simulink model "OMAP_ver_MIL10"  (R2018b)
settings: Solver=FixedStepDiscrete  StartTime=0.0  StopTime=10.0  FixedStep=0.01  RelTol=1e-3
undefined symbols (not defined in the file or in its folder): OMAP_Switch_EMS, OMAP_Switch_EPS, OMAP_Switch_ESC, OMAP_Switch_IC, OMAP_Switch_OTHER, TH_HMIClb_tiDgrdIconWarnHiDurT_C, TH_HMIClb_tiDgrdIconWarnLoDurT_C, TH_HMIClb_tiDgrdVocWarnDurT_C, TH_HMIClb_tiHndOffTxtWarnT_C, TH_HMIClb_tiHndOffVocWarnT_C, TH_HMIClb_tiSWALimFlgDetT_C, TH_HMIClb_tiTxtLimT_C
libraries: simulink x118
(part 8 of 9)

== system OMAP_ver_MIL10/OMAP_Module/ICA_Direct_G59/ICA_Define/Subsystem1/Dspl/DsplPrcs/Txt/TxtOff ==
  TxtOff_stTHState : Inport
  TxtOff_stLstTHState : Inport  Port=2
  Constant1 : Constant  OutDataTypeStr=uint16
  Constant2 : Constant  Value=0  OutDataTypeStr=uint16
  Hold : Subsystem  TreatAsAtomicUnit=on
  If : If  NumInputs=2  IfExpression=u1 == 0 & u2 ~= 0 & u2 ~= 5  ElseIfExpressions=u1 ~= 0
  Merge : Merge  Inputs=3
  Start : Subsystem  TreatAsAtomicUnit=on
  Stop : Subsystem  TreatAsAtomicUnit=on
  Unit Delay1 : UnitDelay  SampleTime=-1
  TxtOff_stOff : Outport
  wires:
  TxtOff_stTHState/1 -> If/1
  Merge/1 -> Unit Delay1/1, TxtOff_stOff/1
  Start/1(Out1) -> Merge/1
  TxtOff_stLstTHState/1 -> If/2
  Constant1/1 -> Start/1(In1)
  If/1 -> Start/Action
  Constant2/1 -> Stop/1(In1)
  If/2 -> Stop/Action
  Unit Delay1/1 -> Hold/1(In1)
  If/3 -> Hold/Action
  Stop/1(Out1) -> Merge/2
  Hold/1(Out1) -> Merge/3

== system OMAP_ver_MIL10/OMAP_Module/ICA_Direct_G59/ICA_Define/Subsystem1/Dspl/DsplPrcs/Txt/TxtOffToFault ==
  TxtOffToFault_stTHState : Inport
  TxtOffToFault_stLstTHState : Inport  Port=2
  TxtOffToFault_stACCState : Inport  Port=3
  Constant1 : Constant  OutDataTypeStr=uint16
  Constant2 : Constant  Value=0  OutDataTypeStr=uint16
  Hold : Subsystem  TreatAsAtomicUnit=on
  If : If  NumInputs=3  IfExpression=u1 == 5 & u2 == 0 & u3 ~= 15  ElseIfExpressions=u1 ~= 5 | u3 == 15
  Merge : Merge  Inputs=3
  Start : Subsystem  TreatAsAtomicUnit=on
  Stop : Subsystem  TreatAsAtomicUnit=on
  Unit Delay1 : UnitDelay  SampleTime=-1
  TxtOffToFault_stOffToFault : Outport
  wires:
  TxtOffToFault_stTHState/1 -> If/1
  Merge/1 -> Unit Delay1/1, TxtOffToFault_stOffToFault/1
  Start/1(Out1) -> Merge/1
  TxtOffToFault_stLstTHState/1 -> If/2
  TxtOffToFault_stACCState/1 -> If/3
  Constant1/1 -> Start/1(In1)
  If/1 -> Start/Action
  Constant2/1 -> Stop/1(In1)
  If/2 -> Stop/Action
  Unit Delay1/1 -> Hold/1(In1)
  If/3 -> Hold/Action
  Stop/1(Out1) -> Merge/2
  Hold/1(Out1) -> Merge/3

== system OMAP_ver_MIL10/OMAP_Module/ICA_Direct_G59/ICA_Define/Subsystem1/Dspl/DsplPrcs/Txt/TxtOn ==
  TxtOn_stTHState : Inport
  TxtOn_stLstTHState : Inport  Port=2
  Constant1 : Constant  OutDataTypeStr=uint16
  Constant2 : Constant  Value=0  OutDataTypeStr=uint16
  Hold : Subsystem  TreatAsAtomicUnit=on
  If : If  NumInputs=2  IfExpression=u1 == 8 & u2 == 0  ElseIfExpressions=u1 == 0 | u1 == 5
  Merge : Merge  Inputs=3
  Start : Subsystem  TreatAsAtomicUnit=on
  Stop : Subsystem  TreatAsAtomicUnit=on
  Unit Delay1 : UnitDelay  SampleTime=-1
  TxtOn_stOn : Outport
  wires:
  TxtOn_stTHState/1 -> If/1
  Merge/1 -> Unit Delay1/1, TxtOn_stOn/1
  Start/1(Out1) -> Merge/1
  TxtOn_stLstTHState/1 -> If/2
  Constant1/1 -> Start/1(In1)
  If/1 -> Start/Action
  Constant2/1 -> Stop/1(In1)
  If/2 -> Stop/Action
  Unit Delay1/1 -> Hold/1(In1)
  If/3 -> Hold/Action
  Stop/1(Out1) -> Merge/2
  Hold/1(Out1) -> Merge/3

== system OMAP_ver_MIL10/OMAP_Module/ICA_Direct_G59/ICA_Define/Subsystem1/Dspl/DsplPrcs/Txt/TxtOnToFault ==
  TxtOnToFault_stTHState : Inport
  TxtOnToFault_stLstTHState : Inport  Port=2
  Constant1 : Constant  OutDataTypeStr=uint16
  Constant2 : Constant  Value=0  OutDataTypeStr=uint16
  Hold : Subsystem  TreatAsAtomicUnit=on
  If : If  NumInputs=2  IfExpression=u1 == 5 & u2 ~= 0 & u2 ~= 5  ElseIfExpressions=u1 ~= 5
  Merge : Merge  Inputs=3
  Start : Subsystem  TreatAsAtomicUnit=on
  Stop : Subsystem  TreatAsAtomicUnit=on
  Unit Delay1 : UnitDelay  SampleTime=-1
  TxtOnToFault_stOnToFault : Outport
  wires:
  Hold/1(Out1) -> Merge/3
  Stop/1(Out1) -> Merge/2
  If/3 -> Hold/Action
  Unit Delay1/1 -> Hold/1(In1)
  If/2 -> Stop/Action
  Constant2/1 -> Stop/1(In1)
  If/1 -> Start/Action
  Constant1/1 -> Start/1(In1)
  TxtOnToFault_stLstTHState/1 -> If/2
  Start/1(Out1) -> Merge/1
  Merge/1 -> TxtOnToFault_stOnToFault/1, Unit Delay1/1
  TxtOnToFault_stTHState/1 -> If/1

== system OMAP_ver_MIL10/OMAP_Module/ICA_Direct_G59/ICA_Define/Subsystem1/Dspl/DsplPrcs/Txt/Txt_Tlimit ==
  incrcondition : Inport
  maxlimit : Inport  Port=2
  Compare To Constant : simulink/Logic and Bit Operations/Compare To Constant  relop===  const=boolean(1)  OutDataTypeStr=boolean
  Compare To Constant1 : simulink/Logic and Bit Operations/Compare To Constant  relop===  const=uint16(0)  OutDataTypeStr=boolean
  Constant : Constant  Value=0  OutDataTypeStr=uint16
  Constant1 : Constant  Value=0  OutDataTypeStr=uint16
  Constant2 : Constant  OutDataTypeStr=uint16
  Constant4 : Constant  OutDataTypeStr=uint16
  Constant5 : Constant  Value=0  OutDataTypeStr=uint16
  Data Type Conversion3 : DataTypeConversion  OutDataTypeStr=uint16
  Detect Fall Nonpositive : simulink/Logic and Bit Operations/Detect Fall Nonpositive  vinit=0  OutDataTypeStr=boolean
      settings: SourceProductName=Simulink  SourceProductBaseCode=SL
  Detect Rise Positive : simulink/Logic and Bit Operations/Detect Rise Positive  vinit=0  OutDataTypeStr=boolean
  Hold : Subsystem  TreatAsAtomicUnit=on
  If : If  NumInputs=3  IfExpression=u1 == 1  ElseIfExpressions=u2 == 1 | u3 == 1
  Logical Operator : Logic  Operator=OR  AllPortsSameDT=off  OutDataTypeStr=boolean
  Merge : Merge  Inputs=3
  MinMax1 : MinMax  Inputs=2  OutDataTypeStr=uint16  InputSameDT=on
  Relational Operator : RelationalOperator  Operator=<=  OutDataTypeStr=boolean  RndMeth=Nearest
  Start : Subsystem  TreatAsAtomicUnit=on
  Stop : Subsystem  TreatAsAtomicUnit=on
  Sum : Sum  OutDataTypeStr=Inherit: Inherit via back propagation  InputSameDT=on
  Unit Delay : UnitDelay  SampleTime=-1
  Unit Delay1 : UnitDelay  SampleTime=-1
  Unit Delay3 : UnitDelay  SampleTime=-1
  inc switch : Switch  Criteria=u2 ~= 0  Threshold=1  OutDataTypeStr=Inherit: Inherit via back propagation  InputSameDT=on
  reset switch : Switch  Criteria=u2 ~= 0  Threshold=1  OutDataTypeStr=Inherit: Inherit via back propagation  InputSameDT=on
  counter_status : Outport
  counter_reset : Outport  Port=2
  wires:
  Unit Delay/1 -> Sum/2
  maxlimit/1 -> Relational Operator/1, MinMax1/2
  MinMax1/1 -> reset switch/3
  Hold/1(Out1) -> Merge/3
  Unit Delay1/1 -> Hold/1(In1)
  If/3 -> Hold/Action
  Stop/1(Out1) -> Merge/2
  Constant4/1 -> Start/1(In1)
  If/1 -> Start/Action
  Start/1(Out1) -> Merge/1
  If/2 -> Stop/Action
  Constant5/1 -> Stop/1(In1)
  incrcondition/1 -> Detect Rise Positive/1, Detect Fall Nonpositive/1
  Detect Rise Positive/1 -> If/1
  Detect Fall Nonpositive/1 -> If/2
  Sum/1 -> MinMax1/1
  reset switch/1 -> Relational Operator/2, Unit Delay/1
  Constant1/1 -> reset switch/1
  Relational Operator/1 -> Unit Delay3/1
  [reset] -> If/3
  [reset] -> Compare To Constant/1
  Constant2/1 -> inc switch/1
  Constant/1 -> inc switch/3
  inc switch/1 -> Sum/1
  Logical Operator/1 -> reset switch/2
  Data Type Conversion3/1 -> counter_reset/1
  Unit Delay3/1 -> Data Type Conversion3/1, [reset]
  Compare To Constant/1 -> Logical Operator/2
  Merge/1 -> Compare To Constant1/1, counter_status/1, inc switch/2, Unit Delay1/1
  Compare To Constant1/1 -> Logical Operator/1

== system OMAP_ver_MIL10/OMAP_Module/ICA_Direct_G59/ICA_Define/Subsystem1/Dspl/DsplPrcs/Txt/Txt_Tlimit1 ==
  incrcondition : Inport
  maxlimit : Inport  Port=2
  Compare To Constant : simulink/Logic and Bit Operations/Compare To Constant  relop===  const=boolean(1)  OutDataTypeStr=boolean
  Compare To Constant1 : simulink/Logic and Bit Operations/Compare To Constant  relop===  const=uint16(0)  OutDataTypeStr=boolean
  Constant : Constant  Value=0  OutDataTypeStr=uint16
  Constant1 : Constant  Value=0  OutDataTypeStr=uint16
  Constant2 : Constant  OutDataTypeStr=uint16
  Constant4 : Constant  OutDataTypeStr=uint16
  Constant5 : Constant  Value=0  OutDataTypeStr=uint16
  Data Type Conversion3 : DataTypeConversion  OutDataTypeStr=uint16
  Detect Fall Nonpositive : simulink/Logic and Bit Operations/Detect Fall Nonpositive  vinit=0  OutDataTypeStr=boolean
      settings: SourceProductName=Simulink  SourceProductBaseCode=SL
  Detect Rise Positive : simulink/Logic and Bit Operations/Detect Rise Positive  vinit=0  OutDataTypeStr=boolean
  Hold : Subsystem  TreatAsAtomicUnit=on
  If : If  NumInputs=3  IfExpression=u1 == 1  ElseIfExpressions=u2 == 1 | u3 == 1
  Logical Operator : Logic  Operator=OR  AllPortsSameDT=off  OutDataTypeStr=boolean
  Merge : Merge  Inputs=3
  MinMax1 : MinMax  Inputs=2  OutDataTypeStr=uint16  InputSameDT=on
  Relational Operator : RelationalOperator  Operator=<=  OutDataTypeStr=boolean  RndMeth=Nearest
  Start : Subsystem  TreatAsAtomicUnit=on
  Stop : Subsystem  TreatAsAtomicUnit=on
  Sum : Sum  OutDataTypeStr=Inherit: Inherit via back propagation  InputSameDT=on
  Unit Delay : UnitDelay  SampleTime=-1
  Unit Delay1 : UnitDelay  SampleTime=-1
  Unit Delay3 : UnitDelay  SampleTime=-1
  inc switch : Switch  Criteria=u2 ~= 0  Threshold=1  OutDataTypeStr=Inherit: Inherit via back propagation  InputSameDT=on
  reset switch : Switch  Criteria=u2 ~= 0  Threshold=1  OutDataTypeStr=Inherit: Inherit via back propagation  InputSameDT=on
  counter_status : Outport
  counter_reset : Outport  Port=2
  wires:
  Compare To Constant1/1 -> Logical Operator/1
  Merge/1 -> Unit Delay1/1, inc switch/2, counter_status/1, Compare To Constant1/1
  Compare To Constant/1 -> Logical Operator/2
  Unit Delay3/1 -> [reset], Data Type Conversion3/1
  Data Type Conversion3/1 -> counter_reset/1
  Logical Operator/1 -> reset switch/2
  inc switch/1 -> Sum/1
  Constant/1 -> inc switch/3
  Constant2/1 -> inc switch/1
  [reset] -> Compare To Constant/1
  [reset] -> If/3
  Relational Operator/1 -> Unit Delay3/1
  Constant1/1 -> reset switch/1
  reset switch/1 -> Unit Delay/1, Relational Operator/2
  Sum/1 -> MinMax1/1
  Detect Fall Nonpositive/1 -> If/2
  Detect Rise Positive/1 -> If/1
  incrcondition/1 -> Detect Fall Nonpositive/1, Detect Rise Positive/1
  Constant5/1 -> Stop/1(In1)
  If/2 -> Stop/Action
  Start/1(Out1) -> Merge/1
  If/1 -> Start/Action
  Constant4/1 -> Start/1(In1)
  Stop/1(Out1) -> Merge/2
  If/3 -> Hold/Action
  Unit Delay1/1 -> Hold/1(In1)
  Hold/1(Out1) -> Merge/3
  MinMax1/1 -> reset switch/3
  maxlimit/1 -> MinMax1/2, Relational Operator/1
  Unit Delay/1 -> Sum/2

== system OMAP_ver_MIL10/OMAP_Module/ICA_Direct_G59/ICA_Define/Subsystem1/Dspl/DsplPrcs/Txt/Txt_Tlimit2 ==
  incrcondition : Inport
  maxlimit : Inport  Port=2
  Compare To Constant : simulink/Logic and Bit Operations/Compare To Constant  relop===  const=boolean(1)  OutDataTypeStr=boolean
  Compare To Constant1 : simulink/Logic and Bit Operations/Compare To Constant  relop===  const=uint16(0)  OutDataTypeStr=boolean
  Constant : Constant  Value=0  OutDataTypeStr=uint16
  Constant1 : Constant  Value=0  OutDataTypeStr=uint16
  Constant2 : Constant  OutDataTypeStr=uint16
  Constant4 : Constant  OutDataTypeStr=uint16
  Constant5 : Constant  Value=0  OutDataTypeStr=uint16
  Data Type Conversion3 : DataTypeConversion  OutDataTypeStr=uint16
  Detect Fall Nonpositive : simulink/Logic and Bit Operations/Detect Fall Nonpositive  vinit=0  OutDataTypeStr=boolean
      settings: SourceProductName=Simulink  SourceProductBaseCode=SL
  Detect Rise Positive : simulink/Logic and Bit Operations/Detect Rise Positive  vinit=0  OutDataTypeStr=boolean
  Hold : Subsystem  TreatAsAtomicUnit=on
  If : If  NumInputs=3  IfExpression=u1 == 1  ElseIfExpressions=u2 == 1 | u3 == 1
  Logical Operator : Logic  Operator=OR  AllPortsSameDT=off  OutDataTypeStr=boolean
  Merge : Merge  Inputs=3
  MinMax1 : MinMax  Inputs=2  OutDataTypeStr=uint16  InputSameDT=on
  Relational Operator : RelationalOperator  Operator=<=  OutDataTypeStr=boolean  RndMeth=Nearest
  Start : Subsystem  TreatAsAtomicUnit=on
  Stop : Subsystem  TreatAsAtomicUnit=on
  Sum : Sum  OutDataTypeStr=Inherit: Inherit via back propagation  InputSameDT=on
  Unit Delay : UnitDelay  SampleTime=-1
  Unit Delay1 : UnitDelay  SampleTime=-1
  Unit Delay3 : UnitDelay  SampleTime=-1
  inc switch : Switch  Criteria=u2 ~= 0  Threshold=1  OutDataTypeStr=Inherit: Inherit via back propagation  InputSameDT=on
  reset switch : Switch  Criteria=u2 ~= 0  Threshold=1  OutDataTypeStr=Inherit: Inherit via back propagation  InputSameDT=on
  counter_status : Outport
  counter_reset : Outport  Port=2
  wires:
  Unit Delay/1 -> Sum/2
  maxlimit/1 -> Relational Operator/1, MinMax1/2
  MinMax1/1 -> reset switch/3
  Hold/1(Out1) -> Merge/3
  Unit Delay1/1 -> Hold/1(In1)
  If/3 -> Hold/Action
  Stop/1(Out1) -> Merge/2
  Constant4/1 -> Start/1(In1)
  If/1 -> Start/Action
  Start/1(Out1) -> Merge/1
  If/2 -> Stop/Action
  Constant5/1 -> Stop/1(In1)
  incrcondition/1 -> Detect Rise Positive/1, Detect Fall Nonpositive/1
  Detect Rise Positive/1 -> If/1
  Detect Fall Nonpositive/1 -> If/2
  Sum/1 -> MinMax1/1
  reset switch/1 -> Relational Operator/2, Unit Delay/1
  Constant1/1 -> reset switch/1
  Relational Operator/1 -> Unit Delay3/1
  [reset] -> If/3
  [reset] -> Compare To Constant/1
  Constant2/1 -> inc switch/1
  Constant/1 -> inc switch/3
  inc switch/1 -> Sum/1
  Logical Operator/1 -> reset switch/2
  Data Type Conversion3/1 -> counter_reset/1
  Unit Delay3/1 -> Data Type Conversion3/1, [reset]
  Compare To Constant/1 -> Logical Operator/2
  Merge/1 -> Compare To Constant1/1, counter_status/1, inc switch/2, Unit Delay1/1
  Compare To Constant1/1 -> Logical Operator/1

== system OMAP_ver_MIL10/OMAP_Module/ICA_Direct_G59/ICA_Define/Subsystem1/Dspl/DsplPrcs/Txt/Txt_Tlimit3 ==
  incrcondition : Inport
  maxlimit : Inport  Port=2
  Compare To Constant : simulink/Logic and Bit Operations/Compare To Constant  relop===  const=boolean(1)  OutDataTypeStr=boolean
  Compare To Constant1 : simulink/Logic and Bit Operations/Compare To Constant  relop===  const=uint16(0)  OutDataTypeStr=boolean
  Constant : Constant  Value=0  OutDataTypeStr=uint16
  Constant1 : Constant  Value=0  OutDataTypeStr=uint16
  Constant2 : Constant  OutDataTypeStr=uint16
  Constant4 : Constant  OutDataTypeStr=uint16
  Constant5 : Constant  Value=0  OutDataTypeStr=uint16
  Data Type Conversion3 : DataTypeConversion  OutDataTypeStr=uint16
  Detect Fall Nonpositive : simulink/Logic and Bit Operations/Detect Fall Nonpositive  vinit=0  OutDataTypeStr=boolean
      settings: SourceProductName=Simulink  SourceProductBaseCode=SL
  Detect Rise Positive : simulink/Logic and Bit Operations/Detect Rise Positive  vinit=0  OutDataTypeStr=boolean
  Hold : Subsystem  TreatAsAtomicUnit=on
  If : If  NumInputs=3  IfExpression=u1 == 1  ElseIfExpressions=u2 == 1 | u3 == 1
  Logical Operator : Logic  Operator=OR  AllPortsSameDT=off  OutDataTypeStr=boolean
  Merge : Merge  Inputs=3
  MinMax1 : MinMax  Inputs=2  OutDataTypeStr=uint16  InputSameDT=on
  Relational Operator : RelationalOperator  Operator=<=  OutDataTypeStr=boolean  RndMeth=Nearest
  Start : Subsystem  TreatAsAtomicUnit=on
  Stop : Subsystem  TreatAsAtomicUnit=on
  Sum : Sum  OutDataTypeStr=Inherit: Inherit via back propagation  InputSameDT=on
  Unit Delay : UnitDelay  SampleTime=-1
  Unit Delay1 : UnitDelay  SampleTime=-1
  Unit Delay3 : UnitDelay  SampleTime=-1
  inc switch : Switch  Criteria=u2 ~= 0  Threshold=1  OutDataTypeStr=Inherit: Inherit via back propagation  InputSameDT=on
  reset switch : Switch  Criteria=u2 ~= 0  Threshold=1  OutDataTypeStr=Inherit: Inherit via back propagation  InputSameDT=on
  counter_status : Outport
  counter_reset : Outport  Port=2
  wires:
  Compare To Constant1/1 -> Logical Operator/1
  Merge/1 -> Unit Delay1/1, inc switch/2, counter_status/1, Compare To Constant1/1
  Compare To Constant/1 -> Logical Operator/2
  Unit Delay3/1 -> [reset], Data Type Conversion3/1
  Data Type Conversion3/1 -> counter_reset/1
  Logical Operator/1 -> reset switch/2
  inc switch/1 -> Sum/1
  Constant/1 -> inc switch/3
  Constant2/1 -> inc switch/1
  [reset] -> Compare To Constant/1
  [reset] -> If/3
  Relational Operator/1 -> Unit Delay3/1
  Constant1/1 -> reset switch/1
  reset switch/1 -> Unit Delay/1, Relational Operator/2
  Sum/1 -> MinMax1/1
  Detect Fall Nonpositive/1 -> If/2
  Detect Rise Positive/1 -> If/1
  incrcondition/1 -> Detect Fall Nonpositive/1, Detect Rise Positive/1
  Constant5/1 -> Stop/1(In1)
  If/2 -> Stop/Action
  Start/1(Out1) -> Merge/1
  If/1 -> Start/Action
  Constant4/1 -> Start/1(In1)
  Stop/1(Out1) -> Merge/2
  If/3 -> Hold/Action
  Unit Delay1/1 -> Hold/1(In1)
  Hold/1(Out1) -> Merge/3
  MinMax1/1 -> reset switch/3
  maxlimit/1 -> MinMax1/2, Relational Operator/1
  Unit Delay/1 -> Sum/2

== system OMAP_ver_MIL10/OMAP_Module/ICA_Direct_G59/ICA_Define/Subsystem1/Dspl/DsplPrcs/Txt/Txt_Tlimit4 ==
  incrcondition : Inport
  maxlimit : Inport  Port=2
  Compare To Constant : simulink/Logic and Bit Operations/Compare To Constant  relop===  const=boolean(1)  OutDataTypeStr=boolean
  Compare To Constant1 : simulink/Logic and Bit Operations/Compare To Constant  relop===  const=uint16(0)  OutDataTypeStr=boolean
  Constant : Constant  Value=0  OutDataTypeStr=uint16
  Constant1 : Constant  Value=0  OutDataTypeStr=uint16
  Constant2 : Constant  OutDataTypeStr=uint16
  Constant4 : Constant  OutDataTypeStr=uint16
  Constant5 : Constant  Value=0  OutDataTypeStr=uint16
  Data Type Conversion3 : DataTypeConversion  OutDataTypeStr=uint16
  Detect Fall Nonpositive : simulink/Logic and Bit Operations/Detect Fall Nonpositive  vinit=0  OutDataTypeStr=boolean
      settings: SourceProductName=Simulink  SourceProductBaseCode=SL
  Detect Rise Positive : simulink/Logic and Bit Operations/Detect Rise Positive  vinit=0  OutDataTypeStr=boolean
  Hold : Subsystem  TreatAsAtomicUnit=on
  If : If  NumInputs=3  IfExpression=u1 == 1  ElseIfExpressions=u2 == 1 | u3 == 1
  Logical Operator : Logic  Operator=OR  AllPortsSameDT=off  OutDataTypeStr=boolean
  Merge : Merge  Inputs=3
  MinMax1 : MinMax  Inputs=2  OutDataTypeStr=uint16  InputSameDT=on
  Relational Operator : RelationalOperator  Operator=<=  OutDataTypeStr=boolean  RndMeth=Nearest
  Start : Subsystem  TreatAsAtomicUnit=on
  Stop : Subsystem  TreatAsAtomicUnit=on
  Sum : Sum  OutDataTypeStr=Inherit: Inherit via back propagation  InputSameDT=on
  Unit Delay : UnitDelay  SampleTime=-1
  Unit Delay1 : UnitDelay  SampleTime=-1
  Unit Delay3 : UnitDelay  SampleTime=-1
  inc switch : Switch  Criteria=u2 ~= 0  Threshold=1  OutDataTypeStr=Inherit: Inherit via back propagation  InputSameDT=on
  reset switch : Switch  Criteria=u2 ~= 0  Threshold=1  OutDataTypeStr=Inherit: Inherit via back propagation  InputSameDT=on
  counter_status : Outport
  counter_reset : Outport  Port=2
  wires:
  Unit Delay/1 -> Sum/2
  maxlimit/1 -> Relational Operator/1, MinMax1/2
  MinMax1/1 -> reset switch/3
  Hold/1(Out1) -> Merge/3
  Unit Delay1/1 -> Hold/1(In1)
  If/3 -> Hold/Action
  Stop/1(Out1) -> Merge/2
  Constant4/1 -> Start/1(In1)
  If/1 -> Start/Action
  Start/1(Out1) -> Merge/1
  If/2 -> Stop/Action
  Constant5/1 -> Stop/1(In1)
  incrcondition/1 -> Detect Rise Positive/1, Detect Fall Nonpositive/1
  Detect Rise Positive/1 -> If/1
  Detect Fall Nonpositive/1 -> If/2
  Sum/1 -> MinMax1/1
  reset switch/1 -> Relational Operator/2, Unit Delay/1
  Constant1/1 -> reset switch/1
  Relational Operator/1 -> Unit Delay3/1
  [reset] -> If/3
  [reset] -> Compare To Constant/1
  Constant2/1 -> inc switch/1
  Constant/1 -> inc switch/3
  inc switch/1 -> Sum/1
  Logical Operator/1 -> reset switch/2
  Data Type Conversion3/1 -> counter_reset/1
  Unit Delay3/1 -> Data Type Conversion3/1, [reset]
  Compare To Constant/1 -> Logical Operator/2
  Merge/1 -> Compare To Constant1/1, counter_status/1, inc switch/2, Unit Delay1/1
  Compare To Constant1/1 -> Logical Operator/1

== system OMAP_ver_MIL10/OMAP_Module/ICA_Direct_G59/ICA_Define/Subsystem1/Dspl/DsplPrcs/Txt/Txt_Tlimit5 ==
  incrcondition : Inport
  maxlimit : Inport  Port=2
  Compare To Constant : simulink/Logic and Bit Operations/Compare To Constant  relop===  const=boolean(1)  OutDataTypeStr=boolean
  Compare To Constant1 : simulink/Logic and Bit Operations/Compare To Constant  relop===  const=uint16(0)  OutDataTypeStr=boolean
  Constant : Constant  Value=0  OutDataTypeStr=uint16
  Constant1 : Constant  Value=0  OutDataTypeStr=uint16
  Constant2 : Constant  OutDataTypeStr=uint16
  Constant4 : Constant  OutDataTypeStr=uint16
  Constant5 : Constant  Value=0  OutDataTypeStr=uint16
  Data Type Conversion3 : DataTypeConversion  OutDataTypeStr=uint16
  Detect Fall Nonpositive : simulink/Logic and Bit Operations/Detect Fall Nonpositive  vinit=0  OutDataTypeStr=boolean
      settings: SourceProductName=Simulink  SourceProductBaseCode=SL
  Detect Rise Positive : simulink/Logic and Bit Operations/Detect Rise Positive  vinit=0  OutDataTypeStr=boolean
  Hold : Subsystem  TreatAsAtomicUnit=on
  If : If  NumInputs=3  IfExpression=u1 == 1  ElseIfExpressions=u2 == 1 | u3 == 1
  Logical Operator : Logic  Operator=OR  AllPortsSameDT=off  OutDataTypeStr=boolean
  Merge : Merge  Inputs=3
  MinMax1 : MinMax  Inputs=2  OutDataTypeStr=uint16  InputSameDT=on
  Relational Operator : RelationalOperator  Operator=<=  OutDataTypeStr=boolean  RndMeth=Nearest
  Start : Subsystem  TreatAsAtomicUnit=on
  Stop : Subsystem  TreatAsAtomicUnit=on
  Sum : Sum  OutDataTypeStr=Inherit: Inherit via back propagation  InputSameDT=on
  Unit Delay : UnitDelay  SampleTime=-1
  Unit Delay1 : UnitDelay  SampleTime=-1
  Unit Delay3 : UnitDelay  SampleTime=-1
  inc switch : Switch  Criteria=u2 ~= 0  Threshold=1  OutDataTypeStr=Inherit: Inherit via back propagation  InputSameDT=on
  reset switch : Switch  Criteria=u2 ~= 0  Threshold=1  OutDataTypeStr=Inherit: Inherit via back propagation  InputSameDT=on
  counter_status : Outport
  counter_reset : Outport  Port=2
  wires:
  Compare To Constant1/1 -> Logical Operator/1
  Merge/1 -> Unit Delay1/1, inc switch/2, counter_status/1, Compare To Constant1/1
  Compare To Constant/1 -> Logical Operator/2
  Unit Delay3/1 -> [reset], Data Type Conversion3/1
  Data Type Conversion3/1 -> counter_reset/1
  Logical Operator/1 -> reset switch/2
  inc switch/1 -> Sum/1
  Constant/1 -> inc switch/3
  Constant2/1 -> inc switch/1
  [reset] -> Compare To Constant/1
  [reset] -> If/3
  Relational Operator/1 -> Unit Delay3/1
  Constant1/1 -> reset switch/1
  reset switch/1 -> Unit Delay/1, Relational Operator/2
  Sum/1 -> MinMax1/1
  Detect Fall Nonpositive/1 -> If/2
  Detect Rise Positive/1 -> If/1
  incrcondition/1 -> Detect Fall Nonpositive/1, Detect Rise Positive/1
  Constant5/1 -> Stop/1(In1)
  If/2 -> Stop/Action
  Start/1(Out1) -> Merge/1
  If/1 -> Start/Action
  Constant4/1 -> Start/1(In1)
  Stop/1(Out1) -> Merge/2
  If/3 -> Hold/Action
  Unit Delay1/1 -> Hold/1(In1)
  Hold/1(Out1) -> Merge/3
  MinMax1/1 -> reset switch/3
  maxlimit/1 -> MinMax1/2, Relational Operator/1
  Unit Delay/1 -> Sum/2

== system OMAP_ver_MIL10/OMAP_Module/ICA_Direct_G59/ICA_Define/Subsystem1/Dspl/DsplPrcs/Txt/Txt_Tlimit6 ==
  incrcondition : Inport
  maxlimit : Inport  Port=2
  Compare To Constant : simulink/Logic and Bit Operations/Compare To Constant  relop===  const=boolean(1)  OutDataTypeStr=boolean
  Compare To Constant1 : simulink/Logic and Bit Operations/Compare To Constant  relop===  const=uint16(0)  OutDataTypeStr=boolean
  Constant : Constant  Value=0  OutDataTypeStr=uint16
  Constant1 : Constant  Value=0  OutDataTypeStr=uint16
  Constant2 : Constant  OutDataTypeStr=uint16
  Constant4 : Constant  OutDataTypeStr=uint16
  Constant5 : Constant  Value=0  OutDataTypeStr=uint16
  Data Type Conversion3 : DataTypeConversion  OutDataTypeStr=uint16
  Detect Fall Nonpositive : simulink/Logic and Bit Operations/Detect Fall Nonpositive  vinit=0  OutDataTypeStr=boolean
      settings: SourceProductName=Simulink  SourceProductBaseCode=SL
  Detect Rise Positive : simulink/Logic and Bit Operations/Detect Rise Positive  vinit=0  OutDataTypeStr=boolean
  Hold : Subsystem  TreatAsAtomicUnit=on
  If : If  NumInputs=3  IfExpression=u1 == 1  ElseIfExpressions=u2 == 1 | u3 == 1
  Logical Operator : Logic  Operator=OR  AllPortsSameDT=off  OutDataTypeStr=boolean
  Merge : Merge  Inputs=3
  MinMax1 : MinMax  Inputs=2  OutDataTypeStr=uint16  InputSameDT=on
  Relational Operator : RelationalOperator  Operator=<=  OutDataTypeStr=boolean  RndMeth=Nearest
  Start : Subsystem  TreatAsAtomicUnit=on
  Stop : Subsystem  TreatAsAtomicUnit=on
  Sum : Sum  OutDataTypeStr=Inherit: Inherit via back propagation  InputSameDT=on
  Unit Delay : UnitDelay  SampleTime=-1
  Unit Delay1 : UnitDelay  SampleTime=-1
  Unit Delay3 : UnitDelay  SampleTime=-1
  inc switch : Switch  Criteria=u2 ~= 0  Threshold=1  OutDataTypeStr=Inherit: Inherit via back propagation  InputSameDT=on
  reset switch : Switch  Criteria=u2 ~= 0  Threshold=1  OutDataTypeStr=Inherit: Inherit via back propagation  InputSameDT=on
  counter_status : Outport
  counter_reset : Outport  Port=2
  wires:
  Unit Delay/1 -> Sum/2
  maxlimit/1 -> Relational Operator/1, MinMax1/2
  MinMax1/1 -> reset switch/3
  Hold/1(Out1) -> Merge/3
  Unit Delay1/1 -> Hold/1(In1)
  If/3 -> Hold/Action
  Stop/1(Out1) -> Merge/2
  Constant4/1 -> Start/1(In1)
  If/1 -> Start/Action
  Start/1(Out1) -> Merge/1
  If/2 -> Stop/Action
  Constant5/1 -> Stop/1(In1)
  incrcondition/1 -> Detect Rise Positive/1, Detect Fall Nonpositive/1
  Detect Rise Positive/1 -> If/1
  Detect Fall Nonpositive/1 -> If/2
  Sum/1 -> MinMax1/1
  reset switch/1 -> Relational Operator/2, Unit Delay/1
  Constant1/1 -> reset switch/1
  Relational Operator/1 -> Unit Delay3/1
  [reset] -> If/3
  [reset] -> Compare To Constant/1
  Constant2/1 -> inc switch/1
  Constant/1 -> inc switch/3
  inc switch/1 -> Sum/1
  Logical Operator/1 -> reset switch/2
  Data Type Conversion3/1 -> counter_reset/1
  Unit Delay3/1 -> Data Type Conversion3/1, [reset]
  Compare To Constant/1 -> Logical Operator/2
  Merge/1 -> Compare To Constant1/1, counter_status/1, inc switch/2, Unit Delay1/1
  Compare To Constant1/1 -> Logical Operator/1

== system OMAP_ver_MIL10/OMAP_Module/ICA_Direct_G59/ICA_Define/Subsystem1/Dspl/DsplPrcs/Txt/Txt_Tlimit7 ==
  incrcondition : Inport
  maxlimit : Inport  Port=2
  Compare To Constant : simulink/Logic and Bit Operations/Compare To Constant  relop===  const=boolean(1)  OutDataTypeStr=boolean
  Compare To Constant1 : simulink/Logic and Bit Operations/Compare To Constant  relop===  const=uint16(0)  OutDataTypeStr=boolean
  Constant : Constant  Value=0  OutDataTypeStr=uint16
  Constant1 : Constant  Value=0  OutDataTypeStr=uint16
  Constant2 : Constant  OutDataTypeStr=uint16
  Constant4 : Constant  OutDataTypeStr=uint16
  Constant5 : Constant  Value=0  OutDataTypeStr=uint16
  Data Type Conversion3 : DataTypeConversion  OutDataTypeStr=uint16
  Detect Fall Nonpositive : simulink/Logic and Bit Operations/Detect Fall Nonpositive  vinit=0  OutDataTypeStr=boolean
      settings: SourceProductName=Simulink  SourceProductBaseCode=SL
  Detect Rise Positive : simulink/Logic and Bit Operations/Detect Rise Positive  vinit=0  OutDataTypeStr=boolean
  Hold : Subsystem  TreatAsAtomicUnit=on
  If : If  NumInputs=3  IfExpression=u1 == 1  ElseIfExpressions=u2 == 1 | u3 == 1
  Logical Operator : Logic  Operator=OR  AllPortsSameDT=off  OutDataTypeStr=boolean
  Merge : Merge  Inputs=3
  MinMax1 : MinMax  Inputs=2  OutDataTypeStr=uint16  InputSameDT=on
  Relational Operator : RelationalOperator  Operator=<=  OutDataTypeStr=boolean  RndMeth=Nearest
  Start : Subsystem  TreatAsAtomicUnit=on
  Stop : Subsystem  TreatAsAtomicUnit=on
  Sum : Sum  OutDataTypeStr=Inherit: Inherit via back propagation  InputSameDT=on
  Unit Delay : UnitDelay  SampleTime=-1
  Unit Delay1 : UnitDelay  SampleTime=-1
  Unit Delay3 : UnitDelay  SampleTime=-1
  inc switch : Switch  Criteria=u2 ~= 0  Threshold=1  OutDataTypeStr=Inherit: Inherit via back propagation  InputSameDT=on
  reset switch : Switch  Criteria=u2 ~= 0  Threshold=1  OutDataTypeStr=Inherit: Inherit via back propagation  InputSameDT=on
  counter_status : Outport
  counter_reset : Outport  Port=2
  wires:
  Compare To Constant1/1 -> Logical Operator/1
  Merge/1 -> Unit Delay1/1, inc switch/2, counter_status/1, Compare To Constant1/1
  Compare To Constant/1 -> Logical Operator/2
  Unit Delay3/1 -> [reset], Data Type Conversion3/1
  Data Type Conversion3/1 -> counter_reset/1
  Logical Operator/1 -> reset switch/2
  inc switch/1 -> Sum/1
  Constant/1 -> inc switch/3
  Constant2/1 -> inc switch/1
  [reset] -> Compare To Constant/1
  [reset] -> If/3
  Relational Operator/1 -> Unit Delay3/1
  Constant1/1 -> reset switch/1
  reset switch/1 -> Unit Delay/1, Relational Operator/2
  Sum/1 -> MinMax1/1
  Detect Fall Nonpositive/1 -> If/2
  Detect Rise Positive/1 -> If/1
  incrcondition/1 -> Detect Fall Nonpositive/1, Detect Rise Positive/1
  Constant5/1 -> Stop/1(In1)
  If/2 -> Stop/Action
  Start/1(Out1) -> Merge/1
  If/1 -> Start/Action
  Constant4/1 -> Start/1(In1)
  Stop/1(Out1) -> Merge/2
  If/3 -> Hold/Action
  Unit Delay1/1 -> Hold/1(In1)
  Hold/1(Out1) -> Merge/3
  MinMax1/1 -> reset switch/3
  maxlimit/1 -> MinMax1/2, Relational Operator/1
  Unit Delay/1 -> Sum/2

== system OMAP_ver_MIL10/OMAP_Module/ICA_Direct_G59/ICA_Define/Subsystem1/Dspl/DsplPrcs/Voc/Sum_Condition ==
  In : Inport
  Sum : Inport  Port=2
  Enable : EnablePort  StatesWhenEnabling=reset
  Add1 : Sum  OutDataTypeStr=single
  Data Type Conversion : DataTypeConversion  OutDataTypeStr=uint16
  Memory : Memory  InheritSampleTime=on
  Relational Operator : RelationalOperator  OutDataTypeStr=boolean  RndMeth=Nearest
  Saturation : Saturate  UpperLimit=100000  LowerLimit=0
  Out : Outport  OutputWhenDisabled=reset  InitialOutput=0
  wires:
  Saturation/1 -> Memory/1, Relational Operator/1
  Relational Operator/1 -> Data Type Conversion/1
  Memory/1 -> Add1/2
  Add1/1 -> Saturation/1
  In/1 -> Add1/1
  Sum/1 -> Relational Operator/2
  Data Type Conversion/1 -> Out/1

== system OMAP_ver_MIL10/OMAP_Module/ICA_Direct_G59/ICA_Define/Subsystem1/Dspl/DsplPrcs/Txt/TxtActv/Hold ==
  In1 : Inport
  Action Port : ActionPort
  Out1 : Outport
  wires:
  In1/1 -> Out1/1

== system OMAP_ver_MIL10/OMAP_Module/ICA_Direct_G59/ICA_Define/Subsystem1/Dspl/DsplPrcs/Txt/TxtActv/Start ==
  In1 : Inport
  Action Port : ActionPort
  Out1 : Outport
  wires:
  In1/1 -> Out1/1

== system OMAP_ver_MIL10/OMAP_Module/ICA_Direct_G59/ICA_Define/Subsystem1/Dspl/DsplPrcs/Txt/TxtActv/Stop ==
  In1 : Inport
  Action Port : ActionPort
  Out1 : Outport
  wires:
  In1/1 -> Out1/1

== system OMAP_ver_MIL10/OMAP_Module/ICA_Direct_G59/ICA_Define/Subsystem1/Dspl/DsplPrcs/Txt/TxtCncl/Hold ==
  In1 : Inport
  Action Port : ActionPort
  Out1 : Outport
  wires:
  In1/1 -> Out1/1

== system OMAP_ver_MIL10/OMAP_Module/ICA_Direct_G59/ICA_Define/Subsystem1/Dspl/DsplPrcs/Txt/TxtCncl/Start ==
  In1 : Inport
  Action Port : ActionPort
  Out1 : Outport
  wires:
  In1/1 -> Out1/1

== system OMAP_ver_MIL10/OMAP_Module/ICA_Direct_G59/ICA_Define/Subsystem1/Dspl/DsplPrcs/Txt/TxtCncl/Stop ==
  In1 : Inport
  Action Port : ActionPort
  Out1 : Outport
  wires:
  In1/1 -> Out1/1

== system OMAP_ver_MIL10/OMAP_Module/ICA_Direct_G59/ICA_Define/Subsystem1/Dspl/DsplPrcs/Txt/TxtDegraded/Hold ==
  In1 : Inport
  Action Port : ActionPort
  Out1 : Outport
  wires:
  In1/1 -> Out1/1

== system OMAP_ver_MIL10/OMAP_Module/ICA_Direct_G59/ICA_Define/Subsystem1/Dspl/DsplPrcs/Txt/TxtDegraded/Start ==
  In1 : Inport
  Action Port : ActionPort
  Out1 : Outport
  wires:
  In1/1 -> Out1/1

== system OMAP_ver_MIL10/OMAP_Module/ICA_Direct_G59/ICA_Define/Subsystem1/Dspl/DsplPrcs/Txt/TxtDegraded/Stop ==
  In1 : Inport
  Action Port : ActionPort
  Out1 : Outport
  wires:
  In1/1 -> Out1/1

== system OMAP_ver_MIL10/OMAP_Module/ICA_Direct_G59/ICA_Define/Subsystem1/Dspl/DsplPrcs/Txt/TxtFromACC/Enabled Subsystem ==
  Num : Inport
  Enable : EnablePort  StatesWhenEnabling=reset
  Add : Sum
  Constant : Constant  OutDataTypeStr=single
  Constant1 : Constant  Value=0  OutDataTypeStr=single
  Delay : Delay  DelayLength=1  InitialCondition=0
  Gain : Gain  Gain=2  ParamDataTypeStr=single
  Relational Operator : RelationalOperator  Operator=<=  OutDataTypeStr=boolean  RndMeth=Nearest
  Saturation Dynamic : simulink/Discontinuities/Saturation Dynamic  OutMin=[]  OutMax=[]  OutDataTypeStr=Inherit: Same as second input  OutDataType=fixdt(1, 16)  OutScaling=2^-10  DoSatur=off
  Triger : Outport  OutputWhenDisabled=reset  InitialOutput=single(0)
  wires:
  Constant/1 -> Add/1
  Delay/1 -> Add/2
  Add/1 -> Saturation Dynamic/2
  Saturation Dynamic/1 -> Relational Operator/2, Delay/1
  Constant1/1 -> Saturation Dynamic/3
  Num/1 -> Relational Operator/1, Gain/1
  Gain/1 -> Saturation Dynamic/1
  Relational Operator/1 -> Triger/1

== system OMAP_ver_MIL10/OMAP_Module/ICA_Direct_G59/ICA_Define/Subsystem1/Dspl/DsplPrcs/Txt/TxtFromACC/Hold ==
  In1 : Inport
  Action Port : ActionPort
  Out1 : Outport
  wires:
  In1/1 -> Out1/1

== system OMAP_ver_MIL10/OMAP_Module/ICA_Direct_G59/ICA_Define/Subsystem1/Dspl/DsplPrcs/Txt/TxtFromACC/RdrBlkInhib ==
  RdrBlkInhib_stTHState : Inport
  RdrBlkInhib_stLstTHState : Inport  Port=2
  RdrBlkInhib_stACCTxtDspl : Inport  Port=3
  Constant1 : Constant  OutDataTypeStr=uint16
  Constant2 : Constant  Value=0  OutDataTypeStr=uint16
  If : If  NumInputs=3  IfExpression=u1 == 5 & u2 == 0 & u3 == 2  ElseIfExpressions=u1 ~= 5 | u3 ~= 2
  Inhibit : Subsystem  TreatAsAtomicUnit=on
  Merge : Merge  Inputs=3
  Unit Delay1 : UnitDelay  SampleTime=-1
  hold_last : Subsystem  TreatAsAtomicUnit=on
  not_Inhibit : Subsystem  TreatAsAtomicUnit=on
  RdrBlkInhib_stRdrBlkInhibFlg : Outport
  wires:
  RdrBlkInhib_stTHState/1 -> If/1
  Merge/1 -> Unit Delay1/1, RdrBlkInhib_stRdrBlkInhibFlg/1
  Inhibit/1(Out1) -> Merge/1
  RdrBlkInhib_stLstTHState/1 -> If/2
  RdrBlkInhib_stACCTxtDspl/1 -> If/3
  Constant1/1 -> Inhibit/1(In1)
  If/1 -> Inhibit/Action
  Constant2/1 -> not_Inhibit/1(In1)
  If/2 -> not_Inhibit/Action
  Unit Delay1/1 -> hold_last/1(In1)
  If/3 -> hold_last/Action
  not_Inhibit/1(Out1) -> Merge/2
  hold_last/1(Out1) -> Merge/3

== system OMAP_ver_MIL10/OMAP_Module/ICA_Direct_G59/ICA_Define/Subsystem1/Dspl/DsplPrcs/Txt/TxtFromACC/Start ==
  In1 : Inport
  Action Port : ActionPort
  Out1 : Outport
  wires:
  In1/1 -> Out1/1

== system OMAP_ver_MIL10/OMAP_Module/ICA_Direct_G59/ICA_Define/Subsystem1/Dspl/DsplPrcs/Txt/TxtFromACC/Start1 ==
  In1 : Inport
  Action Port : ActionPort
  Out1 : Outport
  wires:
  In1/1 -> Out1/1

== system OMAP_ver_MIL10/OMAP_Module/ICA_Direct_G59/ICA_Define/Subsystem1/Dspl/DsplPrcs/Txt/TxtFromACC/Start2 ==
  In1 : Inport
  Action Port : ActionPort
  Out1 : Outport
  wires:
  In1/1 -> Out1/1

== system OMAP_ver_MIL10/OMAP_Module/ICA_Direct_G59/ICA_Define/Subsystem1/Dspl/DsplPrcs/Txt/TxtFromACC/Start3 ==
  In1 : Inport
  Action Port : ActionPort
  Out1 : Outport
  wires:
  In1/1 -> Out1/1

== system OMAP_ver_MIL10/OMAP_Module/ICA_Direct_G59/ICA_Define/Subsystem1/Dspl/DsplPrcs/Txt/TxtFromACC/Start4 ==
  In1 : Inport
  Action Port : ActionPort
  Out1 : Outport
  wires:
  In1/1 -> Out1/1

== system OMAP_ver_MIL10/OMAP_Module/ICA_Direct_G59/ICA_Define/Subsystem1/Dspl/DsplPrcs/Txt/TxtFromACC/Stop ==
  In1 : Inport
  Action Port : ActionPort
  Out1 : Outport
  wires:
  In1/1 -> Out1/1

== system OMAP_ver_MIL10/OMAP_Module/ICA_Direct_G59/ICA_Define/Subsystem1/Dspl/DsplPrcs/Txt/TxtFromACC/Stop1 ==
  In1 : Inport
  Action Port : ActionPort
  Out1 : Outport
  wires:
  In1/1 -> Out1/1

== system OMAP_ver_MIL10/OMAP_Module/ICA_Direct_G59/ICA_Define/Subsystem1/Dspl/DsplPrcs/Txt/TxtFromACC/Stop2 ==
  In1 : Inport
  Action Port : ActionPort
  Out1 : Outport
  wires:
  In1/1 -> Out1/1

== system OMAP_ver_MIL10/OMAP_Module/ICA_Direct_G59/ICA_Define/Subsystem1/Dspl/DsplPrcs/Txt/TxtFromACC/Stop3 ==
  In1 : Inport
  Action Port : ActionPort
  Out1 : Outport
  wires:
  In1/1 -> Out1/1

== system OMAP_ver_MIL10/OMAP_Module/ICA_Direct_G59/ICA_Define/Subsystem1/Dspl/DsplPrcs/Txt/TxtFromACC/Stop4 ==
  In1 : Inport
  Action Port : ActionPort
  Out1 : Outport
  wires:
  In1/1 -> Out1/1

== system OMAP_ver_MIL10/OMAP_Module/ICA_Direct_G59/ICA_Define/Subsystem1/Dspl/DsplPrcs/Txt/TxtInactv/Hold ==
  In1 : Inport
  Action Port : ActionPort
  Out1 : Outport
  wires:
  In1/1 -> Out1/1

== system OMAP_ver_MIL10/OMAP_Module/ICA_Direct_G59/ICA_Define/Subsystem1/Dspl/DsplPrcs/Txt/TxtInactv/Start ==
  In1 : Inport
  Action Port : ActionPort
  Out1 : Outport
  wires:
  In1/1 -> Out1/1

== system OMAP_ver_MIL10/OMAP_Module/ICA_Direct_G59/ICA_Define/Subsystem1/Dspl/DsplPrcs/Txt/TxtInactv/Stop ==
  In1 : Inport
  Action Port : ActionPort
  Out1 : Outport
  wires:
  In1/1 -> Out1/1

== system OMAP_ver_MIL10/OMAP_Module/ICA_Direct_G59/ICA_Define/Subsystem1/Dspl/DsplPrcs/Txt/TxtOff/Hold ==
  In1 : Inport
  Action Port : ActionPort
  Out1 : Outport
  wires:
  In1/1 -> Out1/1

== system OMAP_ver_MIL10/OMAP_Module/ICA_Direct_G59/ICA_Define/Subsystem1/Dspl/DsplPrcs/Txt/TxtOff/Start ==
  In1 : Inport
  Action Port : ActionPort
  Out1 : Outport
  wires:
  In1/1 -> Out1/1

== system OMAP_ver_MIL10/OMAP_Module/ICA_Direct_G59/ICA_Define/Subsystem1/Dspl/DsplPrcs/Txt/TxtOff/Stop ==
  In1 : Inport
  Action Port : ActionPort
  Out1 : Outport
  wires:
  In1/1 -> Out1/1

== system OMAP_ver_MIL10/OMAP_Module/ICA_Direct_G59/ICA_Define/Subsystem1/Dspl/DsplPrcs/Txt/TxtOffToFault/Hold ==
  In1 : Inport
  Action Port : ActionPort
  Out1 : Outport
  wires:
  In1/1 -> Out1/1

== system OMAP_ver_MIL10/OMAP_Module/ICA_Direct_G59/ICA_Define/Subsystem1/Dspl/DsplPrcs/Txt/TxtOffToFault/Start ==
  In1 : Inport
  Action Port : ActionPort
  Out1 : Outport
  wires:
  In1/1 -> Out1/1

== system OMAP_ver_MIL10/OMAP_Module/ICA_Direct_G59/ICA_Define/Subsystem1/Dspl/DsplPrcs/Txt/TxtOffToFault/Stop ==
  In1 : Inport
  Action Port : ActionPort
  Out1 : Outport
  wires:
  In1/1 -> Out1/1

== system OMAP_ver_MIL10/OMAP_Module/ICA_Direct_G59/ICA_Define/Subsystem1/Dspl/DsplPrcs/Txt/TxtOn/Hold ==
  In1 : Inport
  Action Port : ActionPort
  Out1 : Outport
  wires:
  In1/1 -> Out1/1

== system OMAP_ver_MIL10/OMAP_Module/ICA_Direct_G59/ICA_Define/Subsystem1/Dspl/DsplPrcs/Txt/TxtOn/Start ==
  In1 : Inport
  Action Port : ActionPort
  Out1 : Outport
  wires:
  In1/1 -> Out1/1

== system OMAP_ver_MIL10/OMAP_Module/ICA_Direct_G59/ICA_Define/Subsystem1/Dspl/DsplPrcs/Txt/TxtOn/Stop ==
  In1 : Inport
  Action Port : ActionPort
  Out1 : Outport
  wires:
  In1/1 -> Out1/1

== system OMAP_ver_MIL10/OMAP_Module/ICA_Direct_G59/ICA_Define/Subsystem1/Dspl/DsplPrcs/Txt/TxtOnToFault/Hold ==
  In1 : Inport
  Action Port : ActionPort
  Out1 : Outport
  wires:
  In1/1 -> Out1/1

== system OMAP_ver_MIL10/OMAP_Module/ICA_Direct_G59/ICA_Define/Subsystem1/Dspl/DsplPrcs/Txt/TxtOnToFault/Start ==
  In1 : Inport
  Action Port : ActionPort
  Out1 : Outport
  wires:
  In1/1 -> Out1/1

== system OMAP_ver_MIL10/OMAP_Module/ICA_Direct_G59/ICA_Define/Subsystem1/Dspl/DsplPrcs/Txt/TxtOnToFault/Stop ==
  In1 : Inport
  Action Port : ActionPort
  Out1 : Outport
  wires:
  In1/1 -> Out1/1

== system OMAP_ver_MIL10/OMAP_Module/ICA_Direct_G59/ICA_Define/Subsystem1/Dspl/DsplPrcs/Txt/Txt_Tlimit/Hold ==
  In1 : Inport
  Action Port : ActionPort
  Out1 : Outport
  wires:
  In1/1 -> Out1/1

== system OMAP_ver_MIL10/OMAP_Module/ICA_Direct_G59/ICA_Define/Subsystem1/Dspl/DsplPrcs/Txt/Txt_Tlimit/Start ==
  In1 : Inport
  Action Port : ActionPort
  Out1 : Outport
  wires:
  In1/1 -> Out1/1

== system OMAP_ver_MIL10/OMAP_Module/ICA_Direct_G59/ICA_Define/Subsystem1/Dspl/DsplPrcs/Txt/Txt_Tlimit/Stop ==
  In1 : Inport
  Action Port : ActionPort
  Out1 : Outport
  wires:
  In1/1 -> Out1/1

== system OMAP_ver_MIL10/OMAP_Module/ICA_Direct_G59/ICA_Define/Subsystem1/Dspl/DsplPrcs/Txt/Txt_Tlimit1/Hold ==
  In1 : Inport
  Action Port : ActionPort
  Out1 : Outport
  wires:
  In1/1 -> Out1/1

== system OMAP_ver_MIL10/OMAP_Module/ICA_Direct_G59/ICA_Define/Subsystem1/Dspl/DsplPrcs/Txt/Txt_Tlimit1/Start ==
  In1 : Inport
  Action Port : ActionPort
  Out1 : Outport
  wires:
  In1/1 -> Out1/1

== system OMAP_ver_MIL10/OMAP_Module/ICA_Direct_G59/ICA_Define/Subsystem1/Dspl/DsplPrcs/Txt/Txt_Tlimit1/Stop ==
  In1 : Inport
  Action Port : ActionPort
  Out1 : Outport
  wires:
  In1/1 -> Out1/1

== system OMAP_ver_MIL10/OMAP_Module/ICA_Direct_G59/ICA_Define/Subsystem1/Dspl/DsplPrcs/Txt/Txt_Tlimit2/Hold ==
  In1 : Inport
  Action Port : ActionPort
  Out1 : Outport
  wires:
  In1/1 -> Out1/1

== system OMAP_ver_MIL10/OMAP_Module/ICA_Direct_G59/ICA_Define/Subsystem1/Dspl/DsplPrcs/Txt/Txt_Tlimit2/Start ==
  In1 : Inport
  Action Port : ActionPort
  Out1 : Outport
  wires:
  In1/1 -> Out1/1

== system OMAP_ver_MIL10/OMAP_Module/ICA_Direct_G59/ICA_Define/Subsystem1/Dspl/DsplPrcs/Txt/Txt_Tlimit2/Stop ==
  In1 : Inport
  Action Port : ActionPort
  Out1 : Outport
  wires:
  In1/1 -> Out1/1

== system OMAP_ver_MIL10/OMAP_Module/ICA_Direct_G59/ICA_Define/Subsystem1/Dspl/DsplPrcs/Txt/Txt_Tlimit3/Hold ==
  In1 : Inport
  Action Port : ActionPort
  Out1 : Outport
  wires:
  In1/1 -> Out1/1

== system OMAP_ver_MIL10/OMAP_Module/ICA_Direct_G59/ICA_Define/Subsystem1/Dspl/DsplPrcs/Txt/Txt_Tlimit3/Start ==
  In1 : Inport
  Action Port : ActionPort
  Out1 : Outport
  wires:
  In1/1 -> Out1/1

== system OMAP_ver_MIL10/OMAP_Module/ICA_Direct_G59/ICA_Define/Subsystem1/Dspl/DsplPrcs/Txt/Txt_Tlimit3/Stop ==
  In1 : Inport
  Action Port : ActionPort
  Out1 : Outport
  wires:
  In1/1 -> Out1/1

== system OMAP_ver_MIL10/OMAP_Module/ICA_Direct_G59/ICA_Define/Subsystem1/Dspl/DsplPrcs/Txt/Txt_Tlimit4/Hold ==
  In1 : Inport
  Action Port : ActionPort
  Out1 : Outport
  wires:
  In1/1 -> Out1/1

== system OMAP_ver_MIL10/OMAP_Module/ICA_Direct_G59/ICA_Define/Subsystem1/Dspl/DsplPrcs/Txt/Txt_Tlimit4/Start ==
  In1 : Inport
  Action Port : ActionPort
  Out1 : Outport
  wires:
  In1/1 -> Out1/1

== system OMAP_ver_MIL10/OMAP_Module/ICA_Direct_G59/ICA_Define/Subsystem1/Dspl/DsplPrcs/Txt/Txt_Tlimit4/Stop ==
  In1 : Inport
  Action Port : ActionPort
  Out1 : Outport
  wires:
  In1/1 -> Out1/1

== system OMAP_ver_MIL10/OMAP_Module/ICA_Direct_G59/ICA_Define/Subsystem1/Dspl/DsplPrcs/Txt/Txt_Tlimit5/Hold ==
  In1 : Inport
  Action Port : ActionPort
  Out1 : Outport
  wires:
  In1/1 -> Out1/1

== system OMAP_ver_MIL10/OMAP_Module/ICA_Direct_G59/ICA_Define/Subsystem1/Dspl/DsplPrcs/Txt/Txt_Tlimit5/Start ==
  In1 : Inport
  Action Port : ActionPort
  Out1 : Outport
  wires:
  In1/1 -> Out1/1

== system OMAP_ver_MIL10/OMAP_Module/ICA_Direct_G59/ICA_Define/Subsystem1/Dspl/DsplPrcs/Txt/Txt_Tlimit5/Stop ==
  In1 : Inport
  Action Port : ActionPort
  Out1 : Outport
  wires:
  In1/1 -> Out1/1

== system OMAP_ver_MIL10/OMAP_Module/ICA_Direct_G59/ICA_Define/Subsystem1/Dspl/DsplPrcs/Txt/Txt_Tlimit6/Hold ==
  In1 : Inport
  Action Port : ActionPort
  Out1 : Outport
  wires:
  In1/1 -> Out1/1

== system OMAP_ver_MIL10/OMAP_Module/ICA_Direct_G59/ICA_Define/Subsystem1/Dspl/DsplPrcs/Txt/Txt_Tlimit6/Start ==
  In1 : Inport
  Action Port : ActionPort
  Out1 : Outport
  wires:
  In1/1 -> Out1/1

== system OMAP_ver_MIL10/OMAP_Module/ICA_Direct_G59/ICA_Define/Subsystem1/Dspl/DsplPrcs/Txt/Txt_Tlimit6/Stop ==
  In1 : Inport
  Action Port : ActionPort
  Out1 : Outport
  wires:
  In1/1 -> Out1/1

== system OMAP_ver_MIL10/OMAP_Module/ICA_Direct_G59/ICA_Define/Subsystem1/Dspl/DsplPrcs/Txt/Txt_Tlimit7/Hold ==
  In1 : Inport
  Action Port : ActionPort
  Out1 : Outport
  wires:
  In1/1 -> Out1/1

== system OMAP_ver_MIL10/OMAP_Module/ICA_Direct_G59/ICA_Define/Subsystem1/Dspl/DsplPrcs/Txt/Txt_Tlimit7/Start ==
  In1 : Inport
  Action Port : ActionPort
  Out1 : Outport
  wires:
  In1/1 -> Out1/1

== system OMAP_ver_MIL10/OMAP_Module/ICA_Direct_G59/ICA_Define/Subsystem1/Dspl/DsplPrcs/Txt/Txt_Tlimit7/Stop ==
  In1 : Inport
  Action Port : ActionPort
  Out1 : Outport
  wires:
  In1/1 -> Out1/1

== system OMAP_ver_MIL10/OMAP_Module/ICA_Direct_G59/ICA_Define/Subsystem1/Dspl/DsplPrcs/Txt/TxtFromACC/RdrBlkInhib/Inhibit ==
  In1 : Inport
  Action Port : ActionPort
  Out1 : Outport
  wires:
  In1/1 -> Out1/1

== system OMAP_ver_MIL10/OMAP_Module/ICA_Direct_G59/ICA_Define/Subsystem1/Dspl/DsplPrcs/Txt/TxtFromACC/RdrBlkInhib/hold_last ==
  In1 : Inport
  Action Port : ActionPort
  Out1 : Outport
  wires:
  In1/1 -> Out1/1

== system OMAP_ver_MIL10/OMAP_Module/ICA_Direct_G59/ICA_Define/Subsystem1/Dspl/DsplPrcs/Txt/TxtFromACC/RdrBlkInhib/not_Inhibit ==
  In1 : Inport
  Action Port : ActionPort
  Out1 : Outport
  wires:
  In1/1 -> Out1/1

== stateflow chart OMAP_ver_MIL10/OMAP_Module/ACCS_Direct/ACCS_Define/ACC_State_Synthesis(ACC_SS)/If Action Subsystem2/Subsystem4/Chart ==
  state Zero
    en:
    RAPPORT=uint8(0);
  state One
    en:
    RAPPORT=uint8(1);
  (default) -> Zero
  Zero -> One : [after(2,tick)]
  One -> Zero : [[after(2,tick)]]
  data: RAPPORT output uint8

== stateflow chart OMAP_ver_MIL10/OMAP_Module/ACCS_Direct/ACCS_Define/ACC_State_Synthesis(ACC_SS)/If Action Subsystem3/Subsystem6/Chart ==
  state Zero
    en:
    RAPPORT=uint8(0);
  state One
    en:
    RAPPORT=uint8(1);
  (default) -> Zero
  Zero -> One : [after(2,tick)]
  One -> Zero : [after(2,tick)]
  data: RAPPORT output uint8

== matlab function OMAP_ver_MIL10/OMAP_Module/ICA_Direct_G59/ICA_Define/ICA_EPS/EPS_Ctr_Disable/MATLAB Function ==
  data: stEPSCtlState input; stEPSCtlCMD output
function stEPSCtlCMD = fcn(stEPSCtlState)
    stEPSCtlCMD=uint16(2);  %select
end

== matlab function OMAP_ver_MIL10/OMAP_Module/ICA_Direct_G59/ICA_Define/ICA_EPS/EPS_Ctr_Enable/MATLAB Function ==
  data: stEPSCtlState input; stEPSCtlCMD output
function stEPSCtlCMD = fcn(stEPSCtlState)
if stEPSCtlState==uint16(0) %unauthorized
    stEPSCtlCMD=uint16(2);  %select
elseif stEPSCtlState==uint16(2) %available
    stEPSCtlCMD=uint16(3);  %authorized
elseif stEPSCtlState==uint16(1) %authorized
    stEPSCtlCMD=uint16(4);  %active
elseif stEPSCtlState==uint16(3) %active
    stEPSCtlCMD=uint16(4);  %active
else
    stEPSCtlCMD=uint16(2);  %select
end

== matlab function OMAP_ver_MIL10/OMAP_Module/ACCS_Direct/ACCS_Define/CIPV_Data ==
  data: IMAPva_d_obj_id input; IMAPva_g_obj_pos_x input; ACCSve_d_CIPV_ID input; CIPV_ID_Longitudinal_Distance output
function CIPV_ID_Longitudinal_Distance = CIPV_Data(IMAPva_d_obj_id, IMAPva_g_obj_pos_x, ACCSve_d_CIPV_ID)
%%依据CIPV_ID求出对应的纵向距离
%分类有目标和无目标
%依据CIPV_ID值求解其在IMAPva_d_obj_id的index
CIPV_ID_Longitudinal_Distance = single(200);

if ACCSve_d_CIPV_ID ~= 0
    for i = 1:40
        if IMAPva_d_obj_id(i) == ACCSve_d_CIPV_ID
            CIPV_ID_Longitudinal_Distance = IMAPva_g_obj_pos_x(i);
        end
    end
end
end

== matlab function OMAP_ver_MIL10/OMAP_Module/ICA_Direct_G59/ICA_Define/Subsystem1/Count1 ==
  data: count_out output
function count_out = fcn()
%#codegen
persistent count;
if isempty(count)
    count=uint16(0);
end
count=count+uint16(1);
if count>=uint16(300)
    count=uint16(0);
end
count_out = count;

== matlab function OMAP_ver_MIL10/OMAP_Module/ICA_Direct_G59/ICA_Define/Subsystem1/Dspl/DsplPrcs/Txt/PrioPrcs ==
  data: HndOffFlg input; GoReqFlg input; THState input; PrioPrcs_TxtDspl output; OffFlg input; TkOvFlg input; ImmdTkOvFlg input; RdrBlkFlg input; OnToFaultFlg input; OffToFaultFlg input; CnclFlg input; OnFlg input; ActvFlg input; InactvFlg input; DegradedFlg input
function PrioPrcs_TxtDspl  = fcn(HndOffFlg,GoReqFlg, THState,OffFlg,TkOvFlg,ImmdTkOvFlg,RdrBlkFlg,OnToFaultFlg,OffToFaultFlg,CnclFlg,OnFlg,ActvFlg,InactvFlg,DegradedFlg)
if (RdrBlkFlg == uint16(1))
       PrioPrcs_TxtDspl = uint16(2);%% Radar Blocked %%
elseif (OnToFaultFlg == uint16(1))
       PrioPrcs_TxtDspl = uint16(3);%% ICA Fault %%
elseif (OffToFaultFlg == uint16(1))
       PrioPrcs_TxtDspl = uint16(3);%% ICA Fault %%
elseif (OffFlg == uint16(1))
       PrioPrcs_TxtDspl = uint16(11);%% ICA OFF %%
elseif (CnclFlg == uint16(1))
       PrioPrcs_TxtDspl = uint16(10);%% ICA Canceled %%
elseif (InactvFlg == uint16(1))
       PrioPrcs_TxtDspl = uint16(4);%% ICA Activation Unsatisfied %%       
elseif (ActvFlg == uint16(1))
       PrioPrcs_TxtDspl = uint16(5);%% ICA Active %%   
elseif (ImmdTkOvFlg == uint16(1))
       PrioPrcs_TxtDspl = uint16(9);%% Please take over the car immediately %%   
elseif (TkOvFlg == uint16(1))
       PrioPrcs_TxtDspl = uint16(7);%% Please take over the car %%   
elseif ((THState ~= uint16(0))&&(THState ~= uint16(5))&&(HndOffFlg == 1))
       PrioPrcs_TxtDspl = uint16(8);%% Please hold the steering wheel %%          
elseif (GoReqFlg == uint16(1))
       PrioPrcs_TxtDspl = uint16(6);%% ICA go request %%          
elseif (OnFlg == uint16(1))
       PrioPrcs_TxtDspl = uint16(1);%% ICA ON %%  
 elseif (DegradedFlg == uint16(1))
       PrioPrcs_TxtDspl = uint16(12);%% ICA degraded %%        
else
       PrioPrcs_TxtDspl = uint16(0);%% No_display %%
end

== matlab function OMAP_ver_MIL10/OMAP_Module/ICA_Direct_G59/ICA_Define/Subsystem1/Dspl/DsplPrcs/Voc/MATLAB_Function ==
  data: Warning_duration input; Warning output; Trigger input
function Warning = fcn(Warning_duration,Trigger)
%#codegen
persistent count;
if isempty(count)
    count=uint16(0);
end
if Trigger==uint16(1)
    count=Warning_duration;
end
if count>=uint16(1)
    count=count-uint16(1);
end
if count==uint16(0)
    Warning=uint16(0);
else
    Warning=uint16(1);
end
end
